simulink model "lookup_nD_TestGen8"  (R2017b)
settings: Solver=FixedStepDiscrete  StartTime=0.0  StopTime=10.0  RelTol=1e-3
undefined symbols (not defined in the file): Block_TestLib, reset
settings Model: Creator=ktrinh  LastModifiedBy=ktrinh
settings DebuggingCC: ParameterOverflowMsg=none

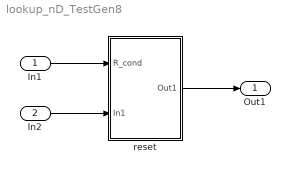
== system lookup_nD_TestGen8 ==
  In1 : Inport
  In2 : Inport  Port=2
  reset : Subsystem  AncestorBlock=Block_TestLib/reset
  Out1 : Outport
  wires:
  In1/1 -> reset/1(R_cond)
  In2/1 -> reset/2(In1)
  reset/1(Out1) -> Out1/1

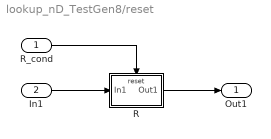
== system lookup_nD_TestGen8/reset ==
  R_cond : Inport  OutDataTypeStr=boolean
  In1 : Inport  Port=2
  R : Subsystem  TreatAsAtomicUnit=on
  Out1 : Outport
  wires:
  R_cond/1 -> R/Reset
  In1/1 -> R/1(In1)
  R/1(Out1) -> Out1/1

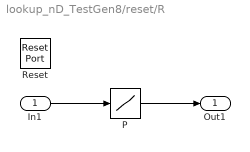
== system lookup_nD_TestGen8/reset/R ==
  In1 : Inport  PortDimensions=2
  Reset : ResetPort  DisableCoverage=on
  P : Lookup_n-D  BreakpointsSpecification=Even spacing  BreakpointsForDimension3=[5, 7]  BreakpointsForDimension1FirstPoint=23.5874  BreakpointsForDimension2FirstPoint=43.5551  BreakpointsForDimension1Spacing=1.5  BreakpointsForDimension2Spacing=1.5  UseOneInputPortForAllInputData=on  Table=[120.511289118853 59.1593020880021 12.2681763288424 85.9903571920136 49.0048148335469;85.8289910062956 84.1633343456099 94.1159437650941 89.9791509510929 6.88697261064177;35.1715539364091 78.9367116880936 108.518066414808 12.2804152272259 100.274056469616]  InterpMethod=Flat  UseLastTableValue=on  InternalRulePriority=Speed  RndMeth=Simplest  InputSameDT=on
  Out1 : Outport
  wires:
  In1/1 -> P/1
  P/1 -> Out1/1
